simulink library "sixdof_model"  (R2021a)
settings: Solver=VariableStepAuto  StartTime=0.0  StopTime=10.0  RelTol=1e-3
settings Model: Creator=prave  LastModifiedBy=prave

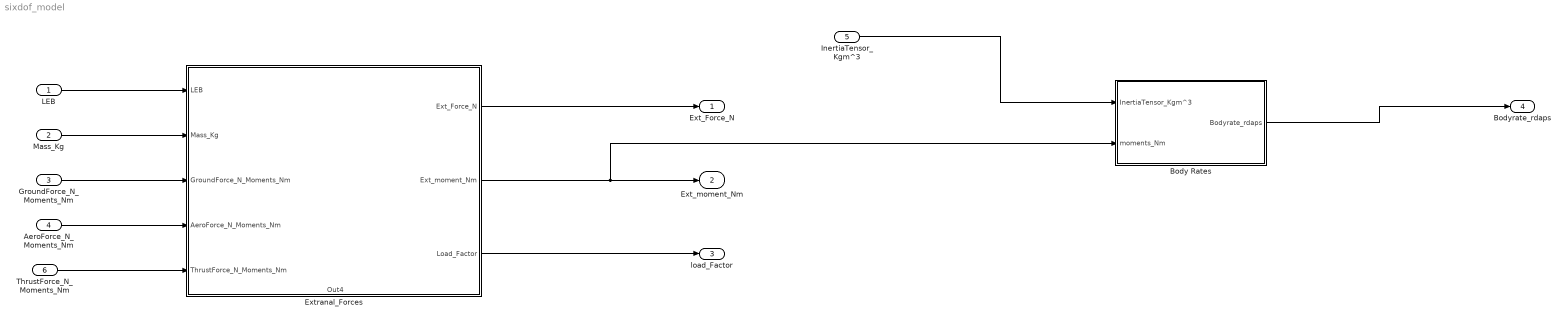
== system sixdof_model ==
  LEB : Inport
  Mass_Kg : Inport  Port=2
  GroundForce_N_Moments_Nm : Inport  Port=3
  AeroForce_N_Moments_Nm : Inport  Port=4
  InertiaTensor_Kgm^3 : Inport  Port=5
  ThrustForce_N_Moments_Nm : Inport  Port=6
  Body Rates : Subsystem
  Extranal_Forces : Subsystem
      settings: PortSchema="{\"entries\":[{\"content\":{\"sides\":[{\"content\":{\"connectorIds\":[\"In1\",\"In2\",\"In3\",\"In4\",\"In5\"]},\"type\":\"ConnectorPlacement.EquallySpacedRectSide\",\"uuid\":\"22d8ea0a-eeda-4b94-a350-540db5d1e472\"},{\"content\":{\"connectorIds\":[\"Out1\",\"Out2\",\"Out3\"],\"side\":\"RIGHT\"},\"type\":\"ConnectorPlacement.EquallySpacedRectSide\",\"uuid\":\"6e76dad5-d25e-441d-8b4a-9e180fb81a8a\"},{\"content\":{\"connectorIds\":[],\"side\":\"TOP\"},\"type\":\"ConnectorPlacement.EquallySpacedRectSide\",\"uuid\":\"7cb076e0-8fb8-4082-98f6-e4b519ad3764\"},{\"content\":{\"connectorIds\":[\"Out4\"],\"side\":\"BOTTOM\"},\"type\":\"ConnectorPlacement.EquallySpacedRectSide\",\"uuid\":\"4be0a506-1c8e-4e29-ab10-4361b8ef561a\"}]},\"type\":\"ConnectorPlacement.EquallySpacedConnector\",\"uuid\":\"ac0412e6-efb0-4aef-af65-18b340b3588e\"}],\"packageUris\":[\"http://schema.mathworks.com/mf0/Connector/R2020b\"],\"version\":\"1.0\"}"
  Ext_Force_N : Outport
  Ext_moment_Nm : Outport  Port=2
  load_Factor : Outport  Port=3
  Bodyrate_rdaps : Outport  Port=4
  wires:
  LEB/1 -> Extranal_Forces/1(LEB)
  Mass_Kg/1 -> Extranal_Forces/2(Mass_Kg)
  GroundForce_N_Moments_Nm/1 -> Extranal_Forces/3(GroundForce_N_Moments_Nm)
  AeroForce_N_Moments_Nm/1 -> Extranal_Forces/4(AeroForce_N_Moments_Nm)
  ThrustForce_N_Moments_Nm/1 -> Extranal_Forces/5(ThrustForce_N_Moments_Nm)
  Extranal_Forces/1(Ext_Force_N) -> Ext_Force_N/1
  Extranal_Forces/3(Load_Factor) -> load_Factor/1
  InertiaTensor_Kgm^3/1 -> Body Rates/1(InertiaTensor_Kgm^3)
  Extranal_Forces/2(Ext_moment_Nm) -> Body Rates/2(moments_Nm), Ext_moment_Nm/1
  Body Rates/1(Bodyrate_rdaps) -> Bodyrate_rdaps/1

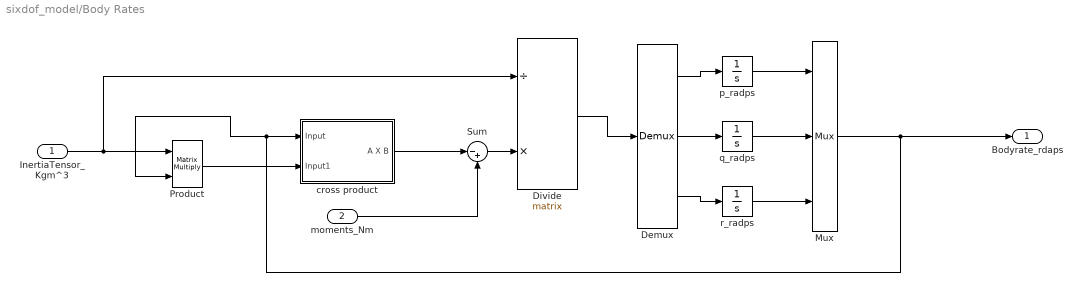
== system sixdof_model/Body Rates ==
  InertiaTensor_Kgm^3 : Inport
  moments_Nm : Inport  Port=2
  Demux : Demux  Outputs=3
  Divide : Product  Inputs=/*  Multiplication=Matrix(*)
  Mux : Mux  Inputs=3
  Product : Product  Multiplication=Matrix(*)
  Sum : Sum  Inputs=|-+
  cross product : Subsystem
  p_radps : Integrator  ContinuousStateAttributes='p_radps'
  q_radps : Integrator  ContinuousStateAttributes='q_radps'
  r_radps : Integrator  ContinuousStateAttributes='r_radps'
  Bodyrate_rdaps : Outport
  wires:
  Demux/2 -> q_radps/1
  Divide/1 -> Demux/1
  Product/1 -> cross product/2(Input1)
  Mux/1 -> Bodyrate_rdaps/1, Product/2, cross product/1(Input)
  cross product/1(A X B) -> Sum/1
  q_radps/1 -> Mux/2
  moments_Nm/1 -> Sum/2
  Demux/1 -> p_radps/1
  InertiaTensor_Kgm^3/1 -> Divide/1, Product/1
  p_radps/1 -> Mux/1
  r_radps/1 -> Mux/3
  Sum/1 -> Divide/2
  Demux/3 -> r_radps/1

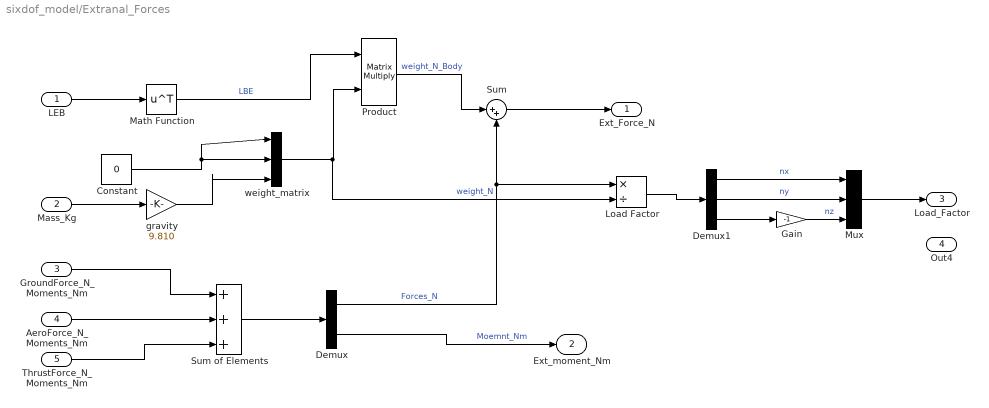
== system sixdof_model/Extranal_Forces ==
  LEB : Inport
  Mass_Kg : Inport  Port=2
  GroundForce_N_Moments_Nm : Inport  Port=3
  AeroForce_N_Moments_Nm : Inport  Port=4
  ThrustForce_N_Moments_Nm : Inport  Port=5
  Constant : Constant  Value=0
  Demux : Demux  Outputs=2
  Demux1 : Demux  Outputs=3
  Gain : Gain  Gain=-1
  Load Factor : Product  Inputs=*/
  Math Function : Math  Operator=transpose  SaturateOnIntegerOverflow=on
  Mux : Mux  Inputs=3
  Product : Product  Multiplication=Matrix(*)
  Sum : Sum  Inputs=|++
  Sum of Elements : Sum  Inputs=+++
  gravity : Gain  Gain=9.810
  weight_matrix : Mux  Inputs=3
  Ext_Force_N : Outport
  Ext_moment_Nm : Outport  Port=2
  Load_Factor : Outport  Port=3
  Out4 : Outport  Port=4
  wires:
  LEB/1 -> Math Function/1
  Product/1 -> Sum/1  "weight_N_Body"
  Mux/1 -> Load_Factor/1
  Demux1/2 -> Mux/2  "ny"
  Constant/1 -> weight_matrix/2, weight_matrix/1
  Demux/1 -> Sum/2, Load Factor/1  "Forces_N"
  GroundForce_N_Moments_Nm/1 -> Sum of Elements/1
  Load Factor/1 -> Demux1/1
  Sum of Elements/1 -> Demux/1
  Demux/2 -> Ext_moment_Nm/1  "Moemnt_Nm"
  weight_matrix/1 -> Load Factor/2, Product/2  "weight_N"
  gravity/1 -> weight_matrix/3
  Sum/1 -> Ext_Force_N/1
  Gain/1 -> Mux/3  "nz"
  Demux1/1 -> Mux/1  "nx"
  Demux1/3 -> Gain/1
  Math Function/1 -> Product/1  "LBE"
  ThrustForce_N_Moments_Nm/1 -> Sum of Elements/3
  AeroForce_N_Moments_Nm/1 -> Sum of Elements/2
  Mass_Kg/1 -> gravity/1

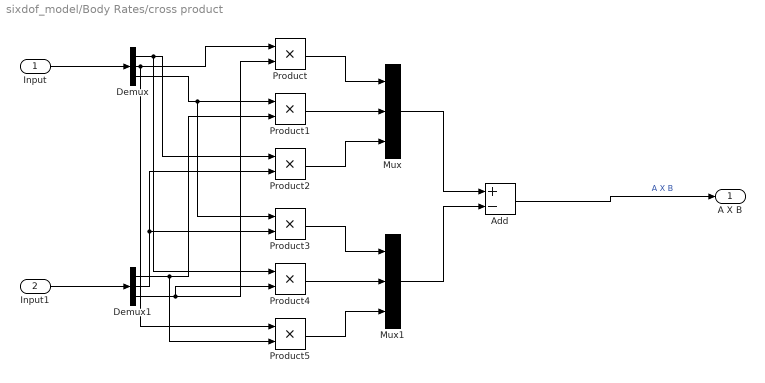
== system sixdof_model/Body Rates/cross product ==
  Input : Inport
  Input1 : Inport  Port=2
  Add : Sum  Inputs=+-
  Demux : Demux  Outputs=3
  Demux1 : Demux  Outputs=3
  Mux : Mux  Inputs=3
  Mux1 : Mux  Inputs=3
  Product{,1..5} (6 alike) : Product
  A X B : Outport
  wires:
  Product/1 -> Mux/1
  Demux1/3 -> Product4/2, Product/2
  Input1/1 -> Demux1/1
  Demux/2 -> Product5/1, Product/1
  Product3/1 -> Mux1/1
  Demux1/1 -> Product5/2, Product1/2
  Demux/3 -> Product3/1, Product1/1
  Demux1/2 -> Product3/2, Product2/2
  Mux/1 -> Add/1
  Product1/1 -> Mux/2
  Product5/1 -> Mux1/3
  Add/1 -> A X B/1  "A X B"
  Product2/1 -> Mux/3
  Product4/1 -> Mux1/2
  Input/1 -> Demux/1
  Demux/1 -> Product4/1, Product2/1
  Mux1/1 -> Add/2
